simulink model "TST_EngPrt_PrtLimOvht"  (R2016b)
settings: Solver=FixedStepDiscrete  StartTime=0.0  StopTime=0.02  FixedStep=sampleTime  RelTol=1e-3
values from neighbouring files (symbols this model uses):
  testCase = 1    [initTST_EngPrt_PrtLimOvht_001.m]    (also in initTST_EngPrt_PrtLimOvht_002.m = 2; initTST_EngPrt_PrtLimOvht_003.m = 3; initTST_EngPrt_PrtLimOvht_004.m = 4; initTST_EngPrt_PrtLimOvht_005.m = 5)
libraries: simulink x21, UnitTest_Lib x10
(part 1 of 2)
settings Model: Creator=zhengjinyan  LastModifiedBy=zhengjinyan
settings DebuggingCC: SignalRangeChecking=error

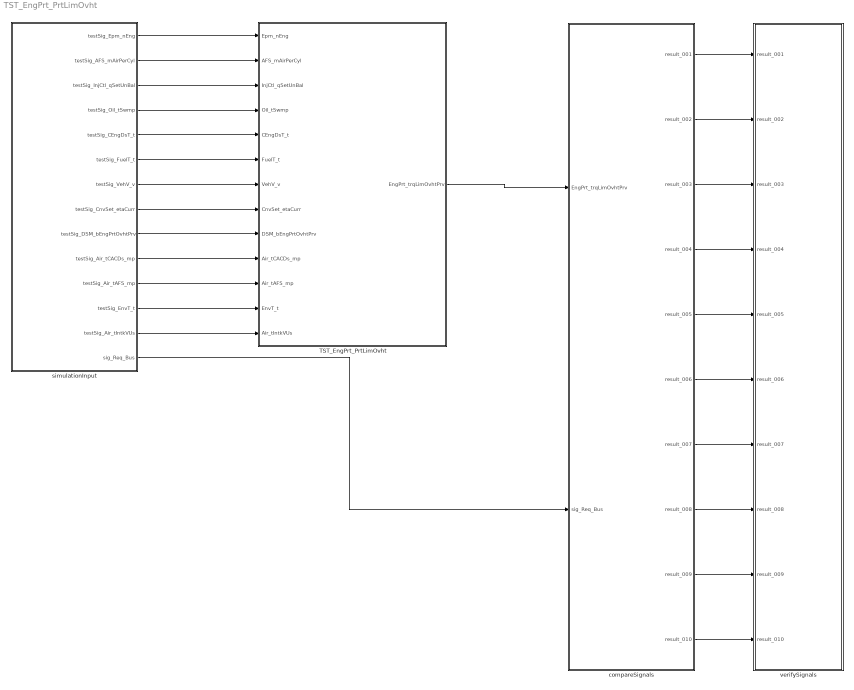
== system TST_EngPrt_PrtLimOvht ==
  TST_EngPrt_PrtLimOvht : Subsystem
  compareSignals : Subsystem
  simulationInput : Subsystem
  verifySignals : Subsystem
  wires:
  simulationInput/1(testSig_Epm_nEng) -> TST_EngPrt_PrtLimOvht/1(Epm_nEng)
  simulationInput/2(testSig_AFS_mAirPerCyl) -> TST_EngPrt_PrtLimOvht/2(AFS_mAirPerCyl)
  simulationInput/3(testSig_InjCtl_qSetUnBal) -> TST_EngPrt_PrtLimOvht/3(InjCtl_qSetUnBal)
  simulationInput/4(testSig_Oil_tSwmp) -> TST_EngPrt_PrtLimOvht/4(Oil_tSwmp)
  simulationInput/5(testSig_CEngDsT_t) -> TST_EngPrt_PrtLimOvht/5(CEngDsT_t)
  simulationInput/6(testSig_FuelT_t) -> TST_EngPrt_PrtLimOvht/6(FuelT_t)
  simulationInput/7(testSig_VehV_v) -> TST_EngPrt_PrtLimOvht/7(VehV_v)
  simulationInput/8(testSig_CnvSet_etaCurr) -> TST_EngPrt_PrtLimOvht/8(CnvSet_etaCurr)
  simulationInput/9(testSig_DSM_bEngPrtOvhtPrv) -> TST_EngPrt_PrtLimOvht/9(DSM_bEngPrtOvhtPrv)
  simulationInput/10(testSig_Air_tCACDs_mp) -> TST_EngPrt_PrtLimOvht/10(Air_tCACDs_mp)
  simulationInput/11(testSig_Air_tAFS_mp) -> TST_EngPrt_PrtLimOvht/11(Air_tAFS_mp)
  simulationInput/12(testSig_EnvT_t) -> TST_EngPrt_PrtLimOvht/12(EnvT_t)
  simulationInput/13(testSig_Air_tIntkVUs) -> TST_EngPrt_PrtLimOvht/13(Air_tIntkVUs)
  TST_EngPrt_PrtLimOvht/1(EngPrt_trqLimOvhtPrv) -> compareSignals/1(EngPrt_trqLimOvhtPrv)
  simulationInput/14(sig_Req_Bus) -> compareSignals/2(sig_Req_Bus)
  compareSignals/1(result_001) -> verifySignals/1(result_001)
  compareSignals/2(result_002) -> verifySignals/2(result_002)
  compareSignals/3(result_003) -> verifySignals/3(result_003)
  compareSignals/4(result_004) -> verifySignals/4(result_004)
  compareSignals/5(result_005) -> verifySignals/5(result_005)
  compareSignals/6(result_006) -> verifySignals/6(result_006)
  compareSignals/7(result_007) -> verifySignals/7(result_007)
  compareSignals/8(result_008) -> verifySignals/8(result_008)
  compareSignals/9(result_009) -> verifySignals/9(result_009)
  compareSignals/10(result_010) -> verifySignals/10(result_010)

== system TST_EngPrt_PrtLimOvht/TST_EngPrt_PrtLimOvht ==
  Epm_nEng : Inport
  AFS_mAirPerCyl : Inport  Port=2
  InjCtl_qSetUnBal : Inport  Port=3
  Oil_tSwmp : Inport  Port=4
  CEngDsT_t : Inport  Port=5
  FuelT_t : Inport  Port=6
  VehV_v : Inport  Port=7
  CnvSet_etaCurr : Inport  Port=8
  DSM_bEngPrtOvhtPrv : Inport  Port=9
  Air_tCACDs_mp : Inport  Port=10
  Air_tAFS_mp : Inport  Port=11
  EnvT_t : Inport  Port=12
  Air_tIntkVUs : Inport  Port=13
  EngPrt_PrtLimOvht : ModelReference  ModelNameDialog=EngPrt_PrtLimOvht  SimulationMode=Normal  ModelReferenceVersion=1.27  TriggerPortName=function  TriggerPortTriggerType=function-call  TriggerPortStatesWhenEnabling=held
  Function_Call : simulink/Ports & Subsystems/Function-Call Generator  sample_time=sampleTime  numberOfIterations=1
  EngPrt_trqLimOvhtPrv : Outport
  wires:
  Function_Call/1 -> EngPrt_PrtLimOvht/Trigger
  Epm_nEng/1 -> EngPrt_PrtLimOvht/1
  AFS_mAirPerCyl/1 -> EngPrt_PrtLimOvht/2
  InjCtl_qSetUnBal/1 -> EngPrt_PrtLimOvht/3
  Oil_tSwmp/1 -> EngPrt_PrtLimOvht/4
  CEngDsT_t/1 -> EngPrt_PrtLimOvht/5
  FuelT_t/1 -> EngPrt_PrtLimOvht/6
  VehV_v/1 -> EngPrt_PrtLimOvht/7
  CnvSet_etaCurr/1 -> EngPrt_PrtLimOvht/8
  DSM_bEngPrtOvhtPrv/1 -> EngPrt_PrtLimOvht/9
  Air_tCACDs_mp/1 -> EngPrt_PrtLimOvht/10
  Air_tAFS_mp/1 -> EngPrt_PrtLimOvht/11
  EnvT_t/1 -> EngPrt_PrtLimOvht/12
  Air_tIntkVUs/1 -> EngPrt_PrtLimOvht/13
  EngPrt_PrtLimOvht/1 -> EngPrt_trqLimOvhtPrv/1

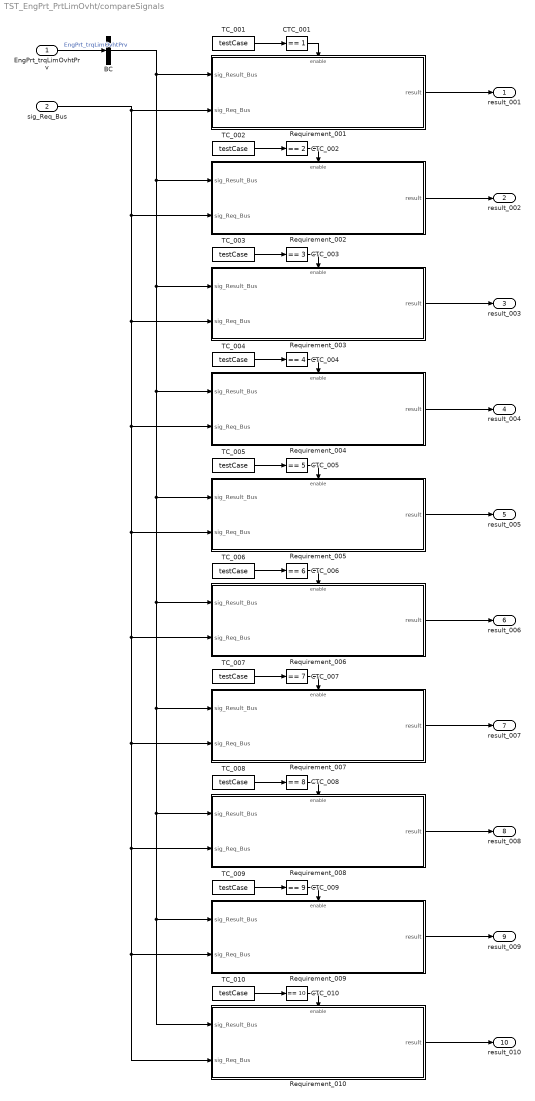
== system TST_EngPrt_PrtLimOvht/compareSignals ==
  EngPrt_trqLimOvhtPrv : Inport
  sig_Req_Bus : Inport  Port=2
  BC : BusCreator  Inputs=1
  CTC_001 : simulink/Logic and Bit Operations/Compare To Constant  relop===  const=1  OutDataTypeStr=boolean
  CTC_002 : simulink/Logic and Bit Operations/Compare To Constant  relop===  const=2  OutDataTypeStr=boolean
  CTC_003 : simulink/Logic and Bit Operations/Compare To Constant  relop===  const=3  OutDataTypeStr=boolean
  CTC_004 : simulink/Logic and Bit Operations/Compare To Constant  relop===  const=4  OutDataTypeStr=boolean
  CTC_005 : simulink/Logic and Bit Operations/Compare To Constant  relop===  const=5  OutDataTypeStr=boolean
  CTC_006 : simulink/Logic and Bit Operations/Compare To Constant  relop===  const=6  OutDataTypeStr=boolean
  CTC_007 : simulink/Logic and Bit Operations/Compare To Constant  relop===  const=7  OutDataTypeStr=boolean
  CTC_008 : simulink/Logic and Bit Operations/Compare To Constant  relop===  const=8  OutDataTypeStr=boolean
  CTC_009 : simulink/Logic and Bit Operations/Compare To Constant  relop===  const=9  OutDataTypeStr=boolean
  CTC_010 : simulink/Logic and Bit Operations/Compare To Constant  relop===  const=10  OutDataTypeStr=boolean
  Requirement_001 : Subsystem
  Requirement_002 : Subsystem
  Requirement_003 : Subsystem
  Requirement_004 : Subsystem
  Requirement_005 : Subsystem
  Requirement_006 : Subsystem
  Requirement_007 : Subsystem
  Requirement_008 : Subsystem
  Requirement_009 : Subsystem
  Requirement_010 : Subsystem
  TC_001 : Constant  Value=testCase
  TC_002 : Constant  Value=testCase
  TC_003 : Constant  Value=testCase
  TC_004 : Constant  Value=testCase
  TC_005 : Constant  Value=testCase
  TC_006 : Constant  Value=testCase
  TC_007 : Constant  Value=testCase
  TC_008 : Constant  Value=testCase
  TC_009 : Constant  Value=testCase
  TC_010 : Constant  Value=testCase
  result_001 : Outport
  result_002 : Outport  Port=2
  result_003 : Outport  Port=3
  result_004 : Outport  Port=4
  result_005 : Outport  Port=5
  result_006 : Outport  Port=6
  result_007 : Outport  Port=7
  result_008 : Outport  Port=8
  result_009 : Outport  Port=9
  result_010 : Outport  Port=10
  wires:
  EngPrt_trqLimOvhtPrv/1 -> BC/1  "EngPrt_trqLimOvhtPrv"
  TC_001/1 -> CTC_001/1
  CTC_001/1 -> Requirement_001/Enable
  sig_Req_Bus/1 -> Requirement_009/2(sig_Req_Bus), Requirement_010/2(sig_Req_Bus), Requirement_008/2(sig_Req_Bus), Requirement_007/2(sig_Req_Bus), Requirement_006/2(sig_Req_Bus), Requirement_005/2(sig_Req_Bus), Requirement_004/2(sig_Req_Bus), Requirement_003/2(sig_Req_Bus), Requirement_002/2(sig_Req_Bus), Requirement_001/2(sig_Req_Bus)
  BC/1 -> Requirement_009/1(sig_Result_Bus), Requirement_010/1(sig_Result_Bus), Requirement_008/1(sig_Result_Bus), Requirement_007/1(sig_Result_Bus), Requirement_006/1(sig_Result_Bus), Requirement_005/1(sig_Result_Bus), Requirement_004/1(sig_Result_Bus), Requirement_003/1(sig_Result_Bus), Requirement_002/1(sig_Result_Bus), Requirement_001/1(sig_Result_Bus)
  Requirement_001/1(result) -> result_001/1
  TC_002/1 -> CTC_002/1
  CTC_002/1 -> Requirement_002/Enable
  Requirement_002/1(result) -> result_002/1
  TC_003/1 -> CTC_003/1
  CTC_003/1 -> Requirement_003/Enable
  Requirement_003/1(result) -> result_003/1
  TC_004/1 -> CTC_004/1
  CTC_004/1 -> Requirement_004/Enable
  Requirement_004/1(result) -> result_004/1
  TC_005/1 -> CTC_005/1
  CTC_005/1 -> Requirement_005/Enable
  Requirement_005/1(result) -> result_005/1
  TC_006/1 -> CTC_006/1
  CTC_006/1 -> Requirement_006/Enable
  Requirement_006/1(result) -> result_006/1
  TC_007/1 -> CTC_007/1
  CTC_007/1 -> Requirement_007/Enable
  Requirement_007/1(result) -> result_007/1
  TC_008/1 -> CTC_008/1
  CTC_008/1 -> Requirement_008/Enable
  Requirement_008/1(result) -> result_008/1
  TC_009/1 -> CTC_009/1
  CTC_009/1 -> Requirement_009/Enable
  Requirement_009/1(result) -> result_009/1
  TC_010/1 -> CTC_010/1
  CTC_010/1 -> Requirement_010/Enable
  Requirement_010/1(result) -> result_010/1

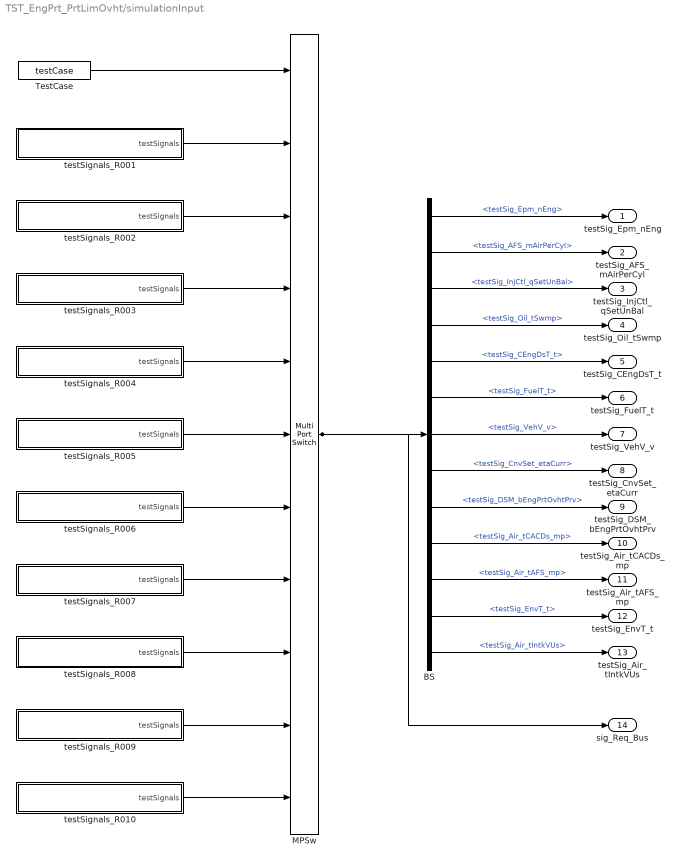
== system TST_EngPrt_PrtLimOvht/simulationInput ==
  BS : BusSelector  OutputSignals=testSig_Epm_nEng,testSig_AFS_mAirPerCyl,testSig_InjCtl_qSetUnBal,testSig_Oil_tSwmp,testSig_CEngDsT_t,testSig_FuelT_t,testSig_VehV_v,testSig_CnvSet_etaCurr,testSig_DSM_bEngPrtOvhtPrv,testSig_Air_tCACDs_mp,testSig_Air_tAFS_mp,testSig_EnvT_t,testSig_Air_tIntkVUs
  MPSw : MultiPortSwitch  Inputs=10  SaturateOnIntegerOverflow=on  InputSameDT=on
  TestCase : Constant  Value=testCase
  testSignals_R001 : Subsystem
  testSignals_R002 : Subsystem
  testSignals_R003 : Subsystem
  testSignals_R004 : Subsystem
  testSignals_R005 : Subsystem
  testSignals_R006 : Subsystem
  testSignals_R007 : Subsystem
  testSignals_R008 : Subsystem
  testSignals_R009 : Subsystem
  testSignals_R010 : Subsystem
  testSig_Epm_nEng : Outport
  testSig_AFS_mAirPerCyl : Outport  Port=2
  testSig_InjCtl_qSetUnBal : Outport  Port=3
  testSig_Oil_tSwmp : Outport  Port=4
  testSig_CEngDsT_t : Outport  Port=5
  testSig_FuelT_t : Outport  Port=6
  testSig_VehV_v : Outport  Port=7
  testSig_CnvSet_etaCurr : Outport  Port=8
  testSig_DSM_bEngPrtOvhtPrv : Outport  Port=9
  testSig_Air_tCACDs_mp : Outport  Port=10
  testSig_Air_tAFS_mp : Outport  Port=11
  testSig_EnvT_t : Outport  Port=12
  testSig_Air_tIntkVUs : Outport  Port=13
  sig_Req_Bus : Outport  Port=14
  wires:
  BS/1 -> testSig_Epm_nEng/1  "<testSig_Epm_nEng>"
  BS/2 -> testSig_AFS_mAirPerCyl/1  "<testSig_AFS_mAirPerCyl>"
  BS/3 -> testSig_InjCtl_qSetUnBal/1  "<testSig_InjCtl_qSetUnBal>"
  BS/4 -> testSig_Oil_tSwmp/1  "<testSig_Oil_tSwmp>"
  BS/5 -> testSig_CEngDsT_t/1  "<testSig_CEngDsT_t>"
  BS/6 -> testSig_FuelT_t/1  "<testSig_FuelT_t>"
  BS/7 -> testSig_VehV_v/1  "<testSig_VehV_v>"
  BS/8 -> testSig_CnvSet_etaCurr/1  "<testSig_CnvSet_etaCurr>"
  BS/9 -> testSig_DSM_bEngPrtOvhtPrv/1  "<testSig_DSM_bEngPrtOvhtPrv>"
  BS/10 -> testSig_Air_tCACDs_mp/1  "<testSig_Air_tCACDs_mp>"
  BS/11 -> testSig_Air_tAFS_mp/1  "<testSig_Air_tAFS_mp>"
  BS/12 -> testSig_EnvT_t/1  "<testSig_EnvT_t>"
  BS/13 -> testSig_Air_tIntkVUs/1  "<testSig_Air_tIntkVUs>"
  MPSw/1 -> BS/1, sig_Req_Bus/1
  TestCase/1 -> MPSw/1
  testSignals_R001/1(testSignals) -> MPSw/2
  testSignals_R002/1(testSignals) -> MPSw/3
  testSignals_R003/1(testSignals) -> MPSw/4
  testSignals_R004/1(testSignals) -> MPSw/5
  testSignals_R005/1(testSignals) -> MPSw/6
  testSignals_R006/1(testSignals) -> MPSw/7
  testSignals_R007/1(testSignals) -> MPSw/8
  testSignals_R008/1(testSignals) -> MPSw/9
  testSignals_R009/1(testSignals) -> MPSw/10
  testSignals_R010/1(testSignals) -> MPSw/11

== system TST_EngPrt_PrtLimOvht/verifySignals ==
  result_001 : Inport
  result_002 : Inport  Port=2
  result_003 : Inport  Port=3
  result_004 : Inport  Port=4
  result_005 : Inport  Port=5
  result_006 : Inport  Port=6
  result_007 : Inport  Port=7
  result_008 : Inport  Port=8
  result_009 : Inport  Port=9
  result_010 : Inport  Port=10
  Assertion_001 : Assertion  Enabled=off
  Assertion_002 : Assertion  Enabled=off
  Assertion_003 : Assertion  Enabled=off
  Assertion_004 : Assertion  Enabled=off
  Assertion_005 : Assertion  Enabled=off
  Assertion_006 : Assertion  Enabled=off
  Assertion_007 : Assertion  Enabled=off
  Assertion_008 : Assertion  Enabled=off
  Assertion_009 : Assertion  Enabled=off
  Assertion_010 : Assertion  Enabled=off
  wires:
  result_001/1 -> Assertion_001/1
  result_002/1 -> Assertion_002/1
  result_003/1 -> Assertion_003/1
  result_004/1 -> Assertion_004/1
  result_005/1 -> Assertion_005/1
  result_006/1 -> Assertion_006/1
  result_007/1 -> Assertion_007/1
  result_008/1 -> Assertion_008/1
  result_009/1 -> Assertion_009/1
  result_010/1 -> Assertion_010/1

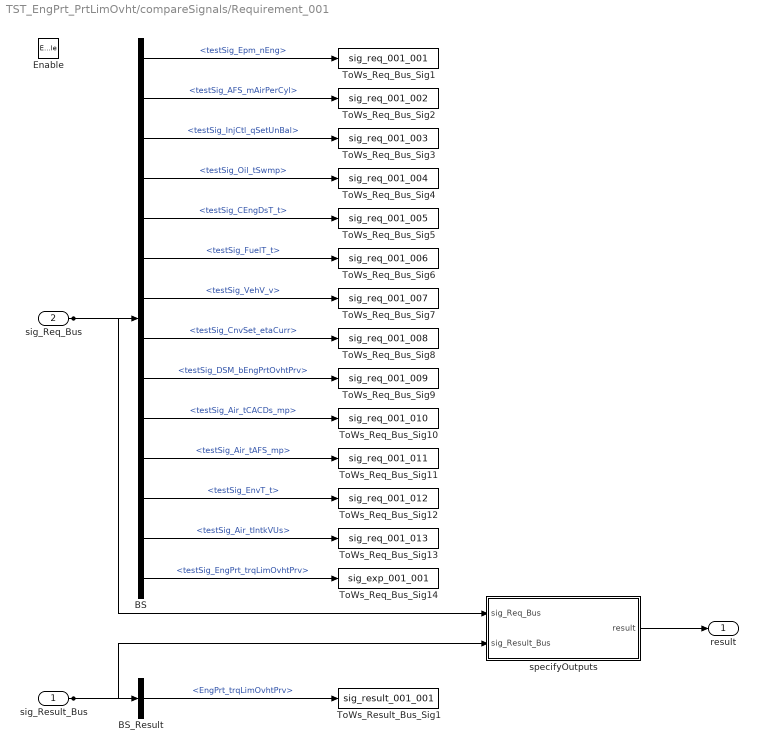
== system TST_EngPrt_PrtLimOvht/compareSignals/Requirement_001 ==
  sig_Result_Bus : Inport
  sig_Req_Bus : Inport  Port=2
  Enable : EnablePort
  BS : BusSelector  OutputSignals=testSig_Epm_nEng,testSig_AFS_mAirPerCyl,testSig_InjCtl_qSetUnBal,testSig_Oil_tSwmp,testSig_CEngDsT_t,testSig_FuelT_t,testSig_VehV_v,testSig_CnvSet_etaCurr,testSig_DSM_bEngPrtOvhtPrv,testSig_Air_tCACDs_mp,testSig_Air_tAFS_mp,testSig_EnvT_t,testSig_Air_tIntkVUs,testSig_EngPrt_trqLimOvhtPrv
  BS_Result : BusSelector  OutputSignals=EngPrt_trqLimOvhtPrv
  ToWs_Req_Bus_Sig1 : ToWorkspace  VariableName=sig_req_001_001  SaveFormat=Structure With Time
  ToWs_Req_Bus_Sig10 : ToWorkspace  VariableName=sig_req_001_010  SaveFormat=Structure With Time
  ToWs_Req_Bus_Sig11 : ToWorkspace  VariableName=sig_req_001_011  SaveFormat=Structure With Time
  ToWs_Req_Bus_Sig12 : ToWorkspace  VariableName=sig_req_001_012  SaveFormat=Structure With Time
  ToWs_Req_Bus_Sig13 : ToWorkspace  VariableName=sig_req_001_013  SaveFormat=Structure With Time
  ToWs_Req_Bus_Sig14 : ToWorkspace  VariableName=sig_exp_001_001  SaveFormat=Structure With Time
  ToWs_Req_Bus_Sig2 : ToWorkspace  VariableName=sig_req_001_002  SaveFormat=Structure With Time
  ToWs_Req_Bus_Sig3 : ToWorkspace  VariableName=sig_req_001_003  SaveFormat=Structure With Time
  ToWs_Req_Bus_Sig4 : ToWorkspace  VariableName=sig_req_001_004  SaveFormat=Structure With Time
  ToWs_Req_Bus_Sig5 : ToWorkspace  VariableName=sig_req_001_005  SaveFormat=Structure With Time
  ToWs_Req_Bus_Sig6 : ToWorkspace  VariableName=sig_req_001_006  SaveFormat=Structure With Time
  ToWs_Req_Bus_Sig7 : ToWorkspace  VariableName=sig_req_001_007  SaveFormat=Structure With Time
  ToWs_Req_Bus_Sig8 : ToWorkspace  VariableName=sig_req_001_008  SaveFormat=Structure With Time
  ToWs_Req_Bus_Sig9 : ToWorkspace  VariableName=sig_req_001_009  SaveFormat=Structure With Time
  ToWs_Result_Bus_Sig1 : ToWorkspace  VariableName=sig_result_001_001  SaveFormat=Structure With Time
  specifyOutputs : Subsystem
  result : Outport
  wires:
  sig_Req_Bus/1 -> BS/1, specifyOutputs/1(sig_Req_Bus)
  BS/1 -> ToWs_Req_Bus_Sig1/1  "<testSig_Epm_nEng>"
  BS/2 -> ToWs_Req_Bus_Sig2/1  "<testSig_AFS_mAirPerCyl>"
  BS/3 -> ToWs_Req_Bus_Sig3/1  "<testSig_InjCtl_qSetUnBal>"
  BS/4 -> ToWs_Req_Bus_Sig4/1  "<testSig_Oil_tSwmp>"
  BS/5 -> ToWs_Req_Bus_Sig5/1  "<testSig_CEngDsT_t>"
  BS/6 -> ToWs_Req_Bus_Sig6/1  "<testSig_FuelT_t>"
  BS/7 -> ToWs_Req_Bus_Sig7/1  "<testSig_VehV_v>"
  BS/8 -> ToWs_Req_Bus_Sig8/1  "<testSig_CnvSet_etaCurr>"
  BS/9 -> ToWs_Req_Bus_Sig9/1  "<testSig_DSM_bEngPrtOvhtPrv>"
  BS/10 -> ToWs_Req_Bus_Sig10/1  "<testSig_Air_tCACDs_mp>"
  BS/11 -> ToWs_Req_Bus_Sig11/1  "<testSig_Air_tAFS_mp>"
  BS/12 -> ToWs_Req_Bus_Sig12/1  "<testSig_EnvT_t>"
  BS/13 -> ToWs_Req_Bus_Sig13/1  "<testSig_Air_tIntkVUs>"
  BS/14 -> ToWs_Req_Bus_Sig14/1  "<testSig_EngPrt_trqLimOvhtPrv>"
  sig_Result_Bus/1 -> BS_Result/1, specifyOutputs/2(sig_Result_Bus)
  BS_Result/1 -> ToWs_Result_Bus_Sig1/1  "<EngPrt_trqLimOvhtPrv>"
  specifyOutputs/1(result) -> result/1

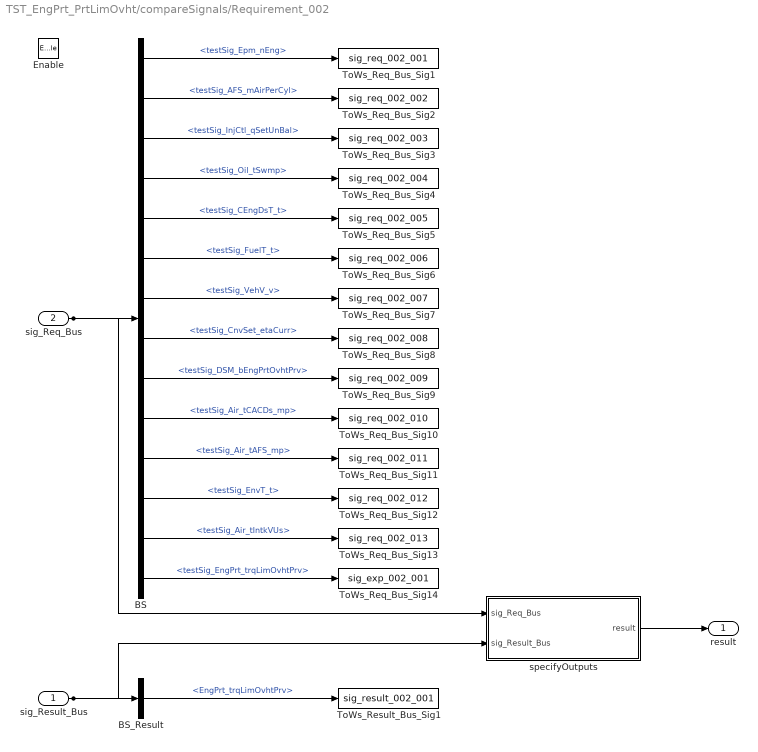
== system TST_EngPrt_PrtLimOvht/compareSignals/Requirement_002 ==
  sig_Result_Bus : Inport
  sig_Req_Bus : Inport  Port=2
  Enable : EnablePort
  BS : BusSelector  OutputSignals=testSig_Epm_nEng,testSig_AFS_mAirPerCyl,testSig_InjCtl_qSetUnBal,testSig_Oil_tSwmp,testSig_CEngDsT_t,testSig_FuelT_t,testSig_VehV_v,testSig_CnvSet_etaCurr,testSig_DSM_bEngPrtOvhtPrv,testSig_Air_tCACDs_mp,testSig_Air_tAFS_mp,testSig_EnvT_t,testSig_Air_tIntkVUs,testSig_EngPrt_trqLimOvhtPrv
  BS_Result : BusSelector  OutputSignals=EngPrt_trqLimOvhtPrv
  ToWs_Req_Bus_Sig1 : ToWorkspace  VariableName=sig_req_002_001  SaveFormat=Structure With Time
  ToWs_Req_Bus_Sig10 : ToWorkspace  VariableName=sig_req_002_010  SaveFormat=Structure With Time
  ToWs_Req_Bus_Sig11 : ToWorkspace  VariableName=sig_req_002_011  SaveFormat=Structure With Time
  ToWs_Req_Bus_Sig12 : ToWorkspace  VariableName=sig_req_002_012  SaveFormat=Structure With Time
  ToWs_Req_Bus_Sig13 : ToWorkspace  VariableName=sig_req_002_013  SaveFormat=Structure With Time
  ToWs_Req_Bus_Sig14 : ToWorkspace  VariableName=sig_exp_002_001  SaveFormat=Structure With Time
  ToWs_Req_Bus_Sig2 : ToWorkspace  VariableName=sig_req_002_002  SaveFormat=Structure With Time
  ToWs_Req_Bus_Sig3 : ToWorkspace  VariableName=sig_req_002_003  SaveFormat=Structure With Time
  ToWs_Req_Bus_Sig4 : ToWorkspace  VariableName=sig_req_002_004  SaveFormat=Structure With Time
  ToWs_Req_Bus_Sig5 : ToWorkspace  VariableName=sig_req_002_005  SaveFormat=Structure With Time
  ToWs_Req_Bus_Sig6 : ToWorkspace  VariableName=sig_req_002_006  SaveFormat=Structure With Time
  ToWs_Req_Bus_Sig7 : ToWorkspace  VariableName=sig_req_002_007  SaveFormat=Structure With Time
  ToWs_Req_Bus_Sig8 : ToWorkspace  VariableName=sig_req_002_008  SaveFormat=Structure With Time
  ToWs_Req_Bus_Sig9 : ToWorkspace  VariableName=sig_req_002_009  SaveFormat=Structure With Time
  ToWs_Result_Bus_Sig1 : ToWorkspace  VariableName=sig_result_002_001  SaveFormat=Structure With Time
  specifyOutputs : Subsystem
  result : Outport
  wires:
  sig_Req_Bus/1 -> BS/1, specifyOutputs/1(sig_Req_Bus)
  BS/1 -> ToWs_Req_Bus_Sig1/1  "<testSig_Epm_nEng>"
  BS/2 -> ToWs_Req_Bus_Sig2/1  "<testSig_AFS_mAirPerCyl>"
  BS/3 -> ToWs_Req_Bus_Sig3/1  "<testSig_InjCtl_qSetUnBal>"
  BS/4 -> ToWs_Req_Bus_Sig4/1  "<testSig_Oil_tSwmp>"
  BS/5 -> ToWs_Req_Bus_Sig5/1  "<testSig_CEngDsT_t>"
  BS/6 -> ToWs_Req_Bus_Sig6/1  "<testSig_FuelT_t>"
  BS/7 -> ToWs_Req_Bus_Sig7/1  "<testSig_VehV_v>"
  BS/8 -> ToWs_Req_Bus_Sig8/1  "<testSig_CnvSet_etaCurr>"
  BS/9 -> ToWs_Req_Bus_Sig9/1  "<testSig_DSM_bEngPrtOvhtPrv>"
  BS/10 -> ToWs_Req_Bus_Sig10/1  "<testSig_Air_tCACDs_mp>"
  BS/11 -> ToWs_Req_Bus_Sig11/1  "<testSig_Air_tAFS_mp>"
  BS/12 -> ToWs_Req_Bus_Sig12/1  "<testSig_EnvT_t>"
  BS/13 -> ToWs_Req_Bus_Sig13/1  "<testSig_Air_tIntkVUs>"
  BS/14 -> ToWs_Req_Bus_Sig14/1  "<testSig_EngPrt_trqLimOvhtPrv>"
  sig_Result_Bus/1 -> BS_Result/1, specifyOutputs/2(sig_Result_Bus)
  BS_Result/1 -> ToWs_Result_Bus_Sig1/1  "<EngPrt_trqLimOvhtPrv>"
  specifyOutputs/1(result) -> result/1

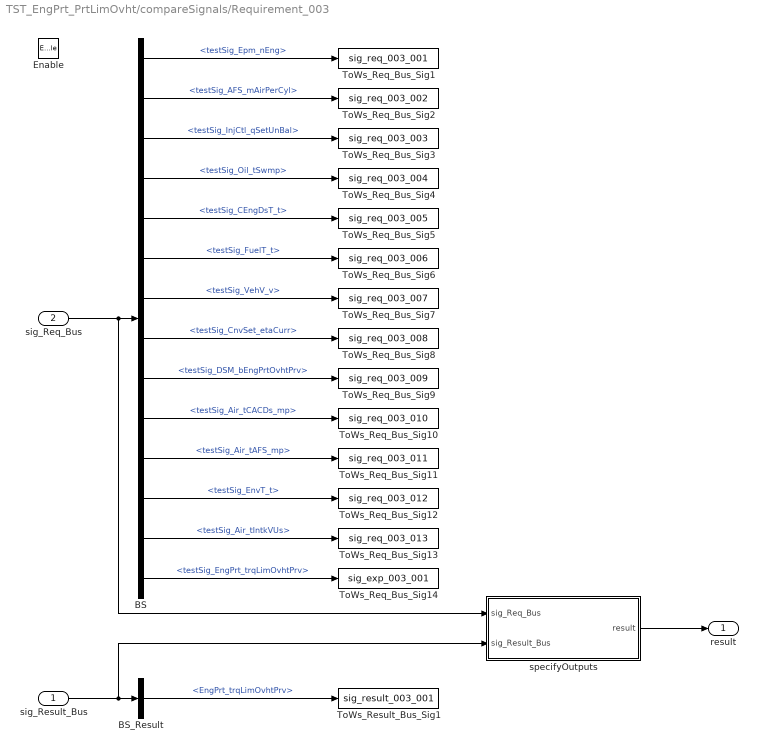
== system TST_EngPrt_PrtLimOvht/compareSignals/Requirement_003 ==
  sig_Result_Bus : Inport
  sig_Req_Bus : Inport  Port=2
  Enable : EnablePort
  BS : BusSelector  OutputSignals=testSig_Epm_nEng,testSig_AFS_mAirPerCyl,testSig_InjCtl_qSetUnBal,testSig_Oil_tSwmp,testSig_CEngDsT_t,testSig_FuelT_t,testSig_VehV_v,testSig_CnvSet_etaCurr,testSig_DSM_bEngPrtOvhtPrv,testSig_Air_tCACDs_mp,testSig_Air_tAFS_mp,testSig_EnvT_t,testSig_Air_tIntkVUs,testSig_EngPrt_trqLimOvhtPrv
  BS_Result : BusSelector  OutputSignals=EngPrt_trqLimOvhtPrv
  ToWs_Req_Bus_Sig1 : ToWorkspace  VariableName=sig_req_003_001  SaveFormat=Structure With Time
  ToWs_Req_Bus_Sig10 : ToWorkspace  VariableName=sig_req_003_010  SaveFormat=Structure With Time
  ToWs_Req_Bus_Sig11 : ToWorkspace  VariableName=sig_req_003_011  SaveFormat=Structure With Time
  ToWs_Req_Bus_Sig12 : ToWorkspace  VariableName=sig_req_003_012  SaveFormat=Structure With Time
  ToWs_Req_Bus_Sig13 : ToWorkspace  VariableName=sig_req_003_013  SaveFormat=Structure With Time
  ToWs_Req_Bus_Sig14 : ToWorkspace  VariableName=sig_exp_003_001  SaveFormat=Structure With Time
  ToWs_Req_Bus_Sig2 : ToWorkspace  VariableName=sig_req_003_002  SaveFormat=Structure With Time
  ToWs_Req_Bus_Sig3 : ToWorkspace  VariableName=sig_req_003_003  SaveFormat=Structure With Time
  ToWs_Req_Bus_Sig4 : ToWorkspace  VariableName=sig_req_003_004  SaveFormat=Structure With Time
  ToWs_Req_Bus_Sig5 : ToWorkspace  VariableName=sig_req_003_005  SaveFormat=Structure With Time
  ToWs_Req_Bus_Sig6 : ToWorkspace  VariableName=sig_req_003_006  SaveFormat=Structure With Time
  ToWs_Req_Bus_Sig7 : ToWorkspace  VariableName=sig_req_003_007  SaveFormat=Structure With Time
  ToWs_Req_Bus_Sig8 : ToWorkspace  VariableName=sig_req_003_008  SaveFormat=Structure With Time
  ToWs_Req_Bus_Sig9 : ToWorkspace  VariableName=sig_req_003_009  SaveFormat=Structure With Time
  ToWs_Result_Bus_Sig1 : ToWorkspace  VariableName=sig_result_003_001  SaveFormat=Structure With Time
  specifyOutputs : Subsystem
  result : Outport
  wires:
  sig_Req_Bus/1 -> BS/1, specifyOutputs/1(sig_Req_Bus)
  BS/1 -> ToWs_Req_Bus_Sig1/1  "<testSig_Epm_nEng>"
  BS/2 -> ToWs_Req_Bus_Sig2/1  "<testSig_AFS_mAirPerCyl>"
  BS/3 -> ToWs_Req_Bus_Sig3/1  "<testSig_InjCtl_qSetUnBal>"
  BS/4 -> ToWs_Req_Bus_Sig4/1  "<testSig_Oil_tSwmp>"
  BS/5 -> ToWs_Req_Bus_Sig5/1  "<testSig_CEngDsT_t>"
  BS/6 -> ToWs_Req_Bus_Sig6/1  "<testSig_FuelT_t>"
  BS/7 -> ToWs_Req_Bus_Sig7/1  "<testSig_VehV_v>"
  BS/8 -> ToWs_Req_Bus_Sig8/1  "<testSig_CnvSet_etaCurr>"
  BS/9 -> ToWs_Req_Bus_Sig9/1  "<testSig_DSM_bEngPrtOvhtPrv>"
  BS/10 -> ToWs_Req_Bus_Sig10/1  "<testSig_Air_tCACDs_mp>"
  BS/11 -> ToWs_Req_Bus_Sig11/1  "<testSig_Air_tAFS_mp>"
  BS/12 -> ToWs_Req_Bus_Sig12/1  "<testSig_EnvT_t>"
  BS/13 -> ToWs_Req_Bus_Sig13/1  "<testSig_Air_tIntkVUs>"
  BS/14 -> ToWs_Req_Bus_Sig14/1  "<testSig_EngPrt_trqLimOvhtPrv>"
  sig_Result_Bus/1 -> BS_Result/1, specifyOutputs/2(sig_Result_Bus)
  BS_Result/1 -> ToWs_Result_Bus_Sig1/1  "<EngPrt_trqLimOvhtPrv>"
  specifyOutputs/1(result) -> result/1

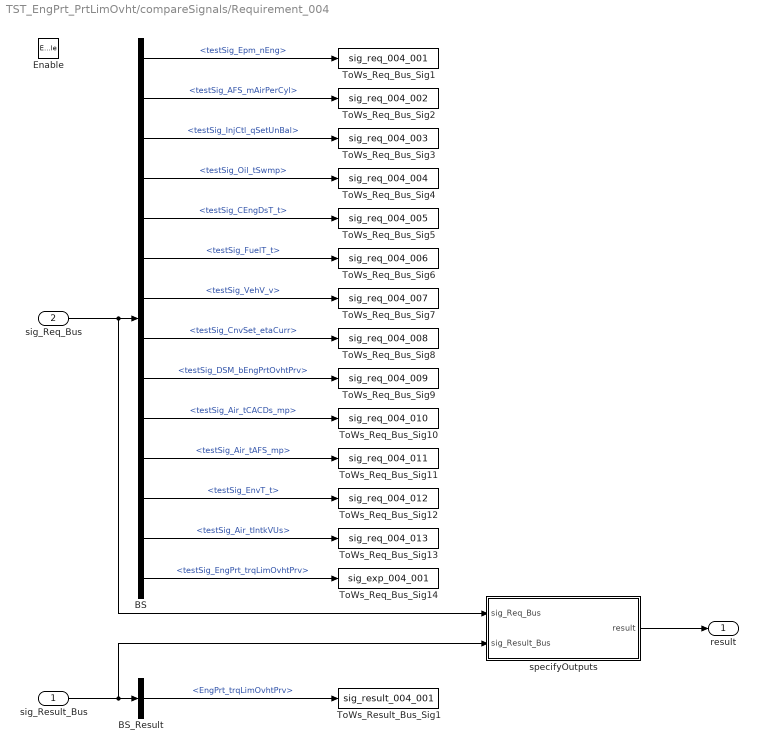
== system TST_EngPrt_PrtLimOvht/compareSignals/Requirement_004 ==
  sig_Result_Bus : Inport
  sig_Req_Bus : Inport  Port=2
  Enable : EnablePort
  BS : BusSelector  OutputSignals=testSig_Epm_nEng,testSig_AFS_mAirPerCyl,testSig_InjCtl_qSetUnBal,testSig_Oil_tSwmp,testSig_CEngDsT_t,testSig_FuelT_t,testSig_VehV_v,testSig_CnvSet_etaCurr,testSig_DSM_bEngPrtOvhtPrv,testSig_Air_tCACDs_mp,testSig_Air_tAFS_mp,testSig_EnvT_t,testSig_Air_tIntkVUs,testSig_EngPrt_trqLimOvhtPrv
  BS_Result : BusSelector  OutputSignals=EngPrt_trqLimOvhtPrv
  ToWs_Req_Bus_Sig1 : ToWorkspace  VariableName=sig_req_004_001  SaveFormat=Structure With Time
  ToWs_Req_Bus_Sig10 : ToWorkspace  VariableName=sig_req_004_010  SaveFormat=Structure With Time
  ToWs_Req_Bus_Sig11 : ToWorkspace  VariableName=sig_req_004_011  SaveFormat=Structure With Time
  ToWs_Req_Bus_Sig12 : ToWorkspace  VariableName=sig_req_004_012  SaveFormat=Structure With Time
  ToWs_Req_Bus_Sig13 : ToWorkspace  VariableName=sig_req_004_013  SaveFormat=Structure With Time
  ToWs_Req_Bus_Sig14 : ToWorkspace  VariableName=sig_exp_004_001  SaveFormat=Structure With Time
  ToWs_Req_Bus_Sig2 : ToWorkspace  VariableName=sig_req_004_002  SaveFormat=Structure With Time
  ToWs_Req_Bus_Sig3 : ToWorkspace  VariableName=sig_req_004_003  SaveFormat=Structure With Time
  ToWs_Req_Bus_Sig4 : ToWorkspace  VariableName=sig_req_004_004  SaveFormat=Structure With Time
  ToWs_Req_Bus_Sig5 : ToWorkspace  VariableName=sig_req_004_005  SaveFormat=Structure With Time
  ToWs_Req_Bus_Sig6 : ToWorkspace  VariableName=sig_req_004_006  SaveFormat=Structure With Time
  ToWs_Req_Bus_Sig7 : ToWorkspace  VariableName=sig_req_004_007  SaveFormat=Structure With Time
  ToWs_Req_Bus_Sig8 : ToWorkspace  VariableName=sig_req_004_008  SaveFormat=Structure With Time
  ToWs_Req_Bus_Sig9 : ToWorkspace  VariableName=sig_req_004_009  SaveFormat=Structure With Time
  ToWs_Result_Bus_Sig1 : ToWorkspace  VariableName=sig_result_004_001  SaveFormat=Structure With Time
  specifyOutputs : Subsystem
  result : Outport
  wires:
  sig_Req_Bus/1 -> BS/1, specifyOutputs/1(sig_Req_Bus)
  BS/1 -> ToWs_Req_Bus_Sig1/1  "<testSig_Epm_nEng>"
  BS/2 -> ToWs_Req_Bus_Sig2/1  "<testSig_AFS_mAirPerCyl>"
  BS/3 -> ToWs_Req_Bus_Sig3/1  "<testSig_InjCtl_qSetUnBal>"
  BS/4 -> ToWs_Req_Bus_Sig4/1  "<testSig_Oil_tSwmp>"
  BS/5 -> ToWs_Req_Bus_Sig5/1  "<testSig_CEngDsT_t>"
  BS/6 -> ToWs_Req_Bus_Sig6/1  "<testSig_FuelT_t>"
  BS/7 -> ToWs_Req_Bus_Sig7/1  "<testSig_VehV_v>"
  BS/8 -> ToWs_Req_Bus_Sig8/1  "<testSig_CnvSet_etaCurr>"
  BS/9 -> ToWs_Req_Bus_Sig9/1  "<testSig_DSM_bEngPrtOvhtPrv>"
  BS/10 -> ToWs_Req_Bus_Sig10/1  "<testSig_Air_tCACDs_mp>"
  BS/11 -> ToWs_Req_Bus_Sig11/1  "<testSig_Air_tAFS_mp>"
  BS/12 -> ToWs_Req_Bus_Sig12/1  "<testSig_EnvT_t>"
  BS/13 -> ToWs_Req_Bus_Sig13/1  "<testSig_Air_tIntkVUs>"
  BS/14 -> ToWs_Req_Bus_Sig14/1  "<testSig_EngPrt_trqLimOvhtPrv>"
  sig_Result_Bus/1 -> BS_Result/1, specifyOutputs/2(sig_Result_Bus)
  BS_Result/1 -> ToWs_Result_Bus_Sig1/1  "<EngPrt_trqLimOvhtPrv>"
  specifyOutputs/1(result) -> result/1

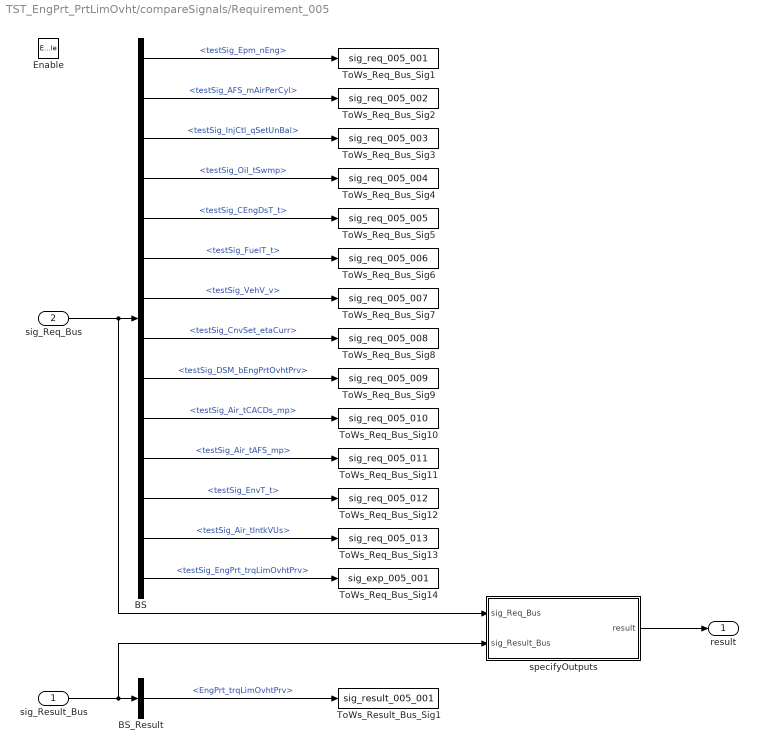
== system TST_EngPrt_PrtLimOvht/compareSignals/Requirement_005 ==
  sig_Result_Bus : Inport
  sig_Req_Bus : Inport  Port=2
  Enable : EnablePort
  BS : BusSelector  OutputSignals=testSig_Epm_nEng,testSig_AFS_mAirPerCyl,testSig_InjCtl_qSetUnBal,testSig_Oil_tSwmp,testSig_CEngDsT_t,testSig_FuelT_t,testSig_VehV_v,testSig_CnvSet_etaCurr,testSig_DSM_bEngPrtOvhtPrv,testSig_Air_tCACDs_mp,testSig_Air_tAFS_mp,testSig_EnvT_t,testSig_Air_tIntkVUs,testSig_EngPrt_trqLimOvhtPrv
  BS_Result : BusSelector  OutputSignals=EngPrt_trqLimOvhtPrv
  ToWs_Req_Bus_Sig1 : ToWorkspace  VariableName=sig_req_005_001  SaveFormat=Structure With Time
  ToWs_Req_Bus_Sig10 : ToWorkspace  VariableName=sig_req_005_010  SaveFormat=Structure With Time
  ToWs_Req_Bus_Sig11 : ToWorkspace  VariableName=sig_req_005_011  SaveFormat=Structure With Time
  ToWs_Req_Bus_Sig12 : ToWorkspace  VariableName=sig_req_005_012  SaveFormat=Structure With Time
  ToWs_Req_Bus_Sig13 : ToWorkspace  VariableName=sig_req_005_013  SaveFormat=Structure With Time
  ToWs_Req_Bus_Sig14 : ToWorkspace  VariableName=sig_exp_005_001  SaveFormat=Structure With Time
  ToWs_Req_Bus_Sig2 : ToWorkspace  VariableName=sig_req_005_002  SaveFormat=Structure With Time
  ToWs_Req_Bus_Sig3 : ToWorkspace  VariableName=sig_req_005_003  SaveFormat=Structure With Time
  ToWs_Req_Bus_Sig4 : ToWorkspace  VariableName=sig_req_005_004  SaveFormat=Structure With Time
  ToWs_Req_Bus_Sig5 : ToWorkspace  VariableName=sig_req_005_005  SaveFormat=Structure With Time
  ToWs_Req_Bus_Sig6 : ToWorkspace  VariableName=sig_req_005_006  SaveFormat=Structure With Time
  ToWs_Req_Bus_Sig7 : ToWorkspace  VariableName=sig_req_005_007  SaveFormat=Structure With Time
  ToWs_Req_Bus_Sig8 : ToWorkspace  VariableName=sig_req_005_008  SaveFormat=Structure With Time
  ToWs_Req_Bus_Sig9 : ToWorkspace  VariableName=sig_req_005_009  SaveFormat=Structure With Time
  ToWs_Result_Bus_Sig1 : ToWorkspace  VariableName=sig_result_005_001  SaveFormat=Structure With Time
  specifyOutputs : Subsystem
  result : Outport
  wires:
  sig_Req_Bus/1 -> BS/1, specifyOutputs/1(sig_Req_Bus)
  BS/1 -> ToWs_Req_Bus_Sig1/1  "<testSig_Epm_nEng>"
  BS/2 -> ToWs_Req_Bus_Sig2/1  "<testSig_AFS_mAirPerCyl>"
  BS/3 -> ToWs_Req_Bus_Sig3/1  "<testSig_InjCtl_qSetUnBal>"
  BS/4 -> ToWs_Req_Bus_Sig4/1  "<testSig_Oil_tSwmp>"
  BS/5 -> ToWs_Req_Bus_Sig5/1  "<testSig_CEngDsT_t>"
  BS/6 -> ToWs_Req_Bus_Sig6/1  "<testSig_FuelT_t>"
  BS/7 -> ToWs_Req_Bus_Sig7/1  "<testSig_VehV_v>"
  BS/8 -> ToWs_Req_Bus_Sig8/1  "<testSig_CnvSet_etaCurr>"
  BS/9 -> ToWs_Req_Bus_Sig9/1  "<testSig_DSM_bEngPrtOvhtPrv>"
  BS/10 -> ToWs_Req_Bus_Sig10/1  "<testSig_Air_tCACDs_mp>"
  BS/11 -> ToWs_Req_Bus_Sig11/1  "<testSig_Air_tAFS_mp>"
  BS/12 -> ToWs_Req_Bus_Sig12/1  "<testSig_EnvT_t>"
  BS/13 -> ToWs_Req_Bus_Sig13/1  "<testSig_Air_tIntkVUs>"
  BS/14 -> ToWs_Req_Bus_Sig14/1  "<testSig_EngPrt_trqLimOvhtPrv>"
  sig_Result_Bus/1 -> BS_Result/1, specifyOutputs/2(sig_Result_Bus)
  BS_Result/1 -> ToWs_Result_Bus_Sig1/1  "<EngPrt_trqLimOvhtPrv>"
  specifyOutputs/1(result) -> result/1

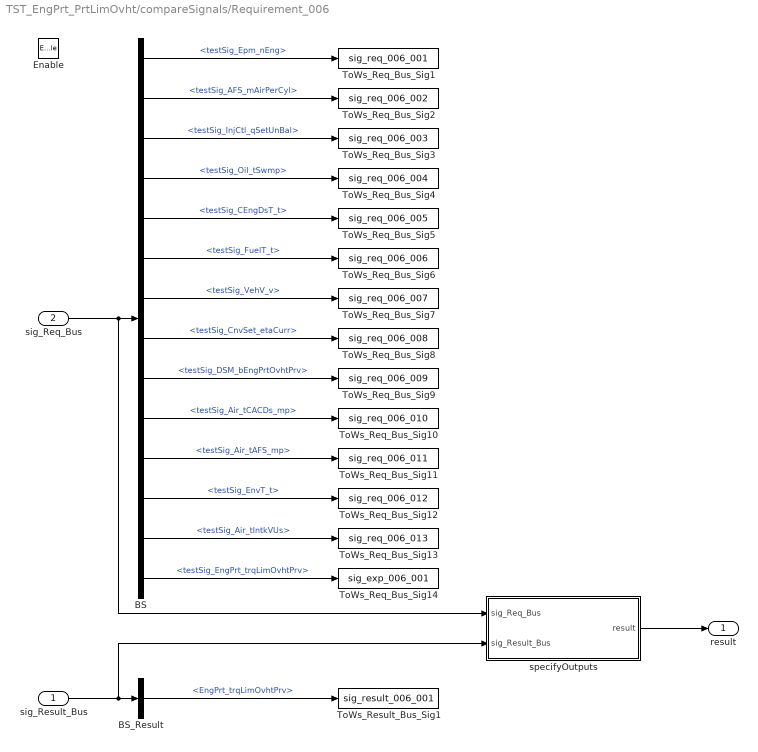
== system TST_EngPrt_PrtLimOvht/compareSignals/Requirement_006 ==
  sig_Result_Bus : Inport
  sig_Req_Bus : Inport  Port=2
  Enable : EnablePort
  BS : BusSelector  OutputSignals=testSig_Epm_nEng,testSig_AFS_mAirPerCyl,testSig_InjCtl_qSetUnBal,testSig_Oil_tSwmp,testSig_CEngDsT_t,testSig_FuelT_t,testSig_VehV_v,testSig_CnvSet_etaCurr,testSig_DSM_bEngPrtOvhtPrv,testSig_Air_tCACDs_mp,testSig_Air_tAFS_mp,testSig_EnvT_t,testSig_Air_tIntkVUs,testSig_EngPrt_trqLimOvhtPrv
  BS_Result : BusSelector  OutputSignals=EngPrt_trqLimOvhtPrv
  ToWs_Req_Bus_Sig1 : ToWorkspace  VariableName=sig_req_006_001  SaveFormat=Structure With Time
  ToWs_Req_Bus_Sig10 : ToWorkspace  VariableName=sig_req_006_010  SaveFormat=Structure With Time
  ToWs_Req_Bus_Sig11 : ToWorkspace  VariableName=sig_req_006_011  SaveFormat=Structure With Time
  ToWs_Req_Bus_Sig12 : ToWorkspace  VariableName=sig_req_006_012  SaveFormat=Structure With Time
  ToWs_Req_Bus_Sig13 : ToWorkspace  VariableName=sig_req_006_013  SaveFormat=Structure With Time
  ToWs_Req_Bus_Sig14 : ToWorkspace  VariableName=sig_exp_006_001  SaveFormat=Structure With Time
  ToWs_Req_Bus_Sig2 : ToWorkspace  VariableName=sig_req_006_002  SaveFormat=Structure With Time
  ToWs_Req_Bus_Sig3 : ToWorkspace  VariableName=sig_req_006_003  SaveFormat=Structure With Time
  ToWs_Req_Bus_Sig4 : ToWorkspace  VariableName=sig_req_006_004  SaveFormat=Structure With Time
  ToWs_Req_Bus_Sig5 : ToWorkspace  VariableName=sig_req_006_005  SaveFormat=Structure With Time
  ToWs_Req_Bus_Sig6 : ToWorkspace  VariableName=sig_req_006_006  SaveFormat=Structure With Time
  ToWs_Req_Bus_Sig7 : ToWorkspace  VariableName=sig_req_006_007  SaveFormat=Structure With Time
  ToWs_Req_Bus_Sig8 : ToWorkspace  VariableName=sig_req_006_008  SaveFormat=Structure With Time
  ToWs_Req_Bus_Sig9 : ToWorkspace  VariableName=sig_req_006_009  SaveFormat=Structure With Time
  ToWs_Result_Bus_Sig1 : ToWorkspace  VariableName=sig_result_006_001  SaveFormat=Structure With Time
  specifyOutputs : Subsystem
  result : Outport
  wires:
  sig_Req_Bus/1 -> BS/1, specifyOutputs/1(sig_Req_Bus)
  BS/1 -> ToWs_Req_Bus_Sig1/1  "<testSig_Epm_nEng>"
  BS/2 -> ToWs_Req_Bus_Sig2/1  "<testSig_AFS_mAirPerCyl>"
  BS/3 -> ToWs_Req_Bus_Sig3/1  "<testSig_InjCtl_qSetUnBal>"
  BS/4 -> ToWs_Req_Bus_Sig4/1  "<testSig_Oil_tSwmp>"
  BS/5 -> ToWs_Req_Bus_Sig5/1  "<testSig_CEngDsT_t>"
  BS/6 -> ToWs_Req_Bus_Sig6/1  "<testSig_FuelT_t>"
  BS/7 -> ToWs_Req_Bus_Sig7/1  "<testSig_VehV_v>"
  BS/8 -> ToWs_Req_Bus_Sig8/1  "<testSig_CnvSet_etaCurr>"
  BS/9 -> ToWs_Req_Bus_Sig9/1  "<testSig_DSM_bEngPrtOvhtPrv>"
  BS/10 -> ToWs_Req_Bus_Sig10/1  "<testSig_Air_tCACDs_mp>"
  BS/11 -> ToWs_Req_Bus_Sig11/1  "<testSig_Air_tAFS_mp>"
  BS/12 -> ToWs_Req_Bus_Sig12/1  "<testSig_EnvT_t>"
  BS/13 -> ToWs_Req_Bus_Sig13/1  "<testSig_Air_tIntkVUs>"
  BS/14 -> ToWs_Req_Bus_Sig14/1  "<testSig_EngPrt_trqLimOvhtPrv>"
  sig_Result_Bus/1 -> BS_Result/1, specifyOutputs/2(sig_Result_Bus)
  BS_Result/1 -> ToWs_Result_Bus_Sig1/1  "<EngPrt_trqLimOvhtPrv>"
  specifyOutputs/1(result) -> result/1

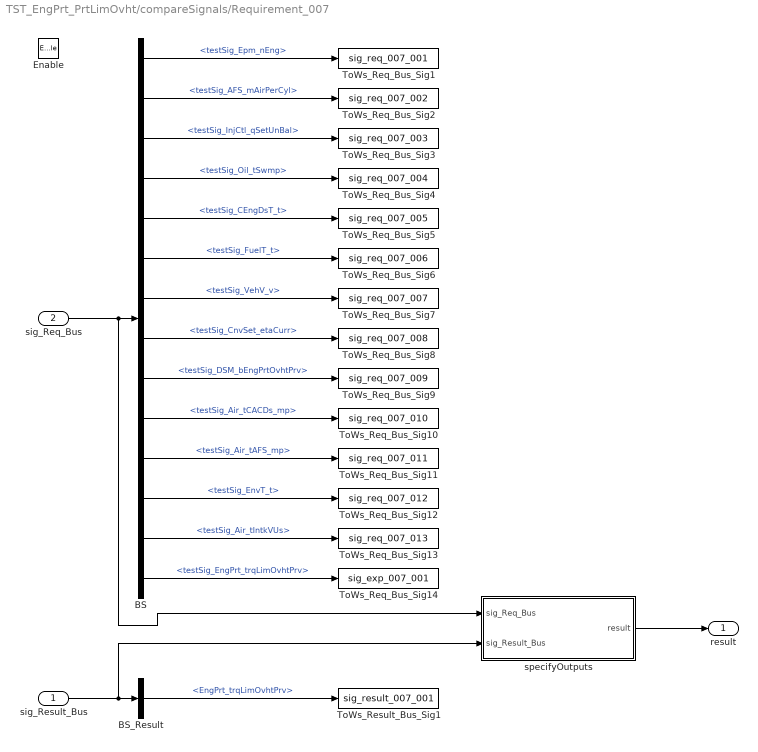
== system TST_EngPrt_PrtLimOvht/compareSignals/Requirement_007 ==
  sig_Result_Bus : Inport
  sig_Req_Bus : Inport  Port=2
  Enable : EnablePort
  BS : BusSelector  OutputSignals=testSig_Epm_nEng,testSig_AFS_mAirPerCyl,testSig_InjCtl_qSetUnBal,testSig_Oil_tSwmp,testSig_CEngDsT_t,testSig_FuelT_t,testSig_VehV_v,testSig_CnvSet_etaCurr,testSig_DSM_bEngPrtOvhtPrv,testSig_Air_tCACDs_mp,testSig_Air_tAFS_mp,testSig_EnvT_t,testSig_Air_tIntkVUs,testSig_EngPrt_trqLimOvhtPrv
  BS_Result : BusSelector  OutputSignals=EngPrt_trqLimOvhtPrv
  ToWs_Req_Bus_Sig1 : ToWorkspace  VariableName=sig_req_007_001  SaveFormat=Structure With Time
  ToWs_Req_Bus_Sig10 : ToWorkspace  VariableName=sig_req_007_010  SaveFormat=Structure With Time
  ToWs_Req_Bus_Sig11 : ToWorkspace  VariableName=sig_req_007_011  SaveFormat=Structure With Time
  ToWs_Req_Bus_Sig12 : ToWorkspace  VariableName=sig_req_007_012  SaveFormat=Structure With Time
  ToWs_Req_Bus_Sig13 : ToWorkspace  VariableName=sig_req_007_013  SaveFormat=Structure With Time
  ToWs_Req_Bus_Sig14 : ToWorkspace  VariableName=sig_exp_007_001  SaveFormat=Structure With Time
  ToWs_Req_Bus_Sig2 : ToWorkspace  VariableName=sig_req_007_002  SaveFormat=Structure With Time
  ToWs_Req_Bus_Sig3 : ToWorkspace  VariableName=sig_req_007_003  SaveFormat=Structure With Time
  ToWs_Req_Bus_Sig4 : ToWorkspace  VariableName=sig_req_007_004  SaveFormat=Structure With Time
  ToWs_Req_Bus_Sig5 : ToWorkspace  VariableName=sig_req_007_005  SaveFormat=Structure With Time
  ToWs_Req_Bus_Sig6 : ToWorkspace  VariableName=sig_req_007_006  SaveFormat=Structure With Time
  ToWs_Req_Bus_Sig7 : ToWorkspace  VariableName=sig_req_007_007  SaveFormat=Structure With Time
  ToWs_Req_Bus_Sig8 : ToWorkspace  VariableName=sig_req_007_008  SaveFormat=Structure With Time
  ToWs_Req_Bus_Sig9 : ToWorkspace  VariableName=sig_req_007_009  SaveFormat=Structure With Time
  ToWs_Result_Bus_Sig1 : ToWorkspace  VariableName=sig_result_007_001  SaveFormat=Structure With Time
  specifyOutputs : Subsystem
  result : Outport
  wires:
  sig_Req_Bus/1 -> BS/1, specifyOutputs/1(sig_Req_Bus)
  BS/1 -> ToWs_Req_Bus_Sig1/1  "<testSig_Epm_nEng>"
  BS/2 -> ToWs_Req_Bus_Sig2/1  "<testSig_AFS_mAirPerCyl>"
  BS/3 -> ToWs_Req_Bus_Sig3/1  "<testSig_InjCtl_qSetUnBal>"
  BS/4 -> ToWs_Req_Bus_Sig4/1  "<testSig_Oil_tSwmp>"
  BS/5 -> ToWs_Req_Bus_Sig5/1  "<testSig_CEngDsT_t>"
  BS/6 -> ToWs_Req_Bus_Sig6/1  "<testSig_FuelT_t>"
  BS/7 -> ToWs_Req_Bus_Sig7/1  "<testSig_VehV_v>"
  BS/8 -> ToWs_Req_Bus_Sig8/1  "<testSig_CnvSet_etaCurr>"
  BS/9 -> ToWs_Req_Bus_Sig9/1  "<testSig_DSM_bEngPrtOvhtPrv>"
  BS/10 -> ToWs_Req_Bus_Sig10/1  "<testSig_Air_tCACDs_mp>"
  BS/11 -> ToWs_Req_Bus_Sig11/1  "<testSig_Air_tAFS_mp>"
  BS/12 -> ToWs_Req_Bus_Sig12/1  "<testSig_EnvT_t>"
  BS/13 -> ToWs_Req_Bus_Sig13/1  "<testSig_Air_tIntkVUs>"
  BS/14 -> ToWs_Req_Bus_Sig14/1  "<testSig_EngPrt_trqLimOvhtPrv>"
  sig_Result_Bus/1 -> BS_Result/1, specifyOutputs/2(sig_Result_Bus)
  BS_Result/1 -> ToWs_Result_Bus_Sig1/1  "<EngPrt_trqLimOvhtPrv>"
  specifyOutputs/1(result) -> result/1

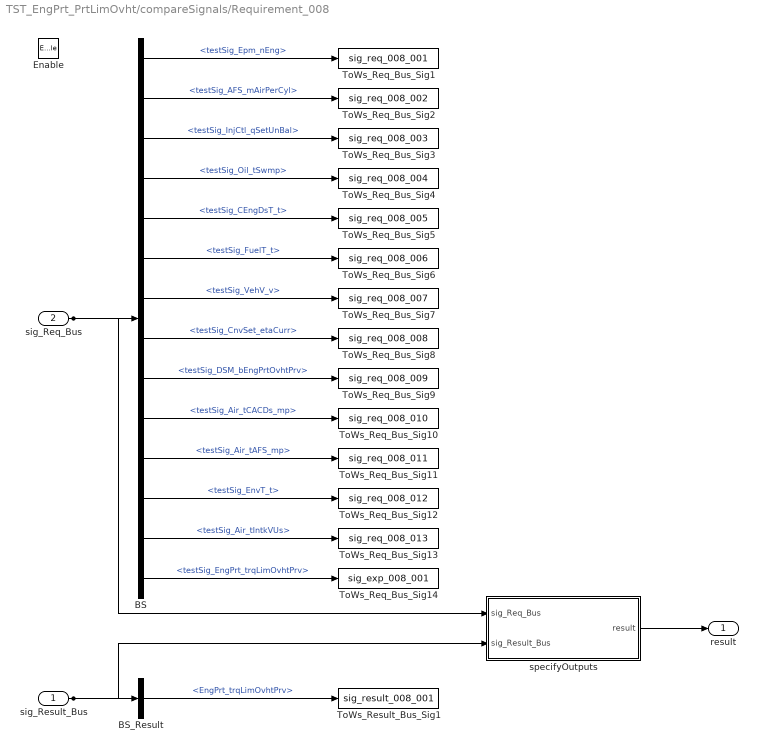
== system TST_EngPrt_PrtLimOvht/compareSignals/Requirement_008 ==
  sig_Result_Bus : Inport
  sig_Req_Bus : Inport  Port=2
  Enable : EnablePort
  BS : BusSelector  OutputSignals=testSig_Epm_nEng,testSig_AFS_mAirPerCyl,testSig_InjCtl_qSetUnBal,testSig_Oil_tSwmp,testSig_CEngDsT_t,testSig_FuelT_t,testSig_VehV_v,testSig_CnvSet_etaCurr,testSig_DSM_bEngPrtOvhtPrv,testSig_Air_tCACDs_mp,testSig_Air_tAFS_mp,testSig_EnvT_t,testSig_Air_tIntkVUs,testSig_EngPrt_trqLimOvhtPrv
  BS_Result : BusSelector  OutputSignals=EngPrt_trqLimOvhtPrv
  ToWs_Req_Bus_Sig1 : ToWorkspace  VariableName=sig_req_008_001  SaveFormat=Structure With Time
  ToWs_Req_Bus_Sig10 : ToWorkspace  VariableName=sig_req_008_010  SaveFormat=Structure With Time
  ToWs_Req_Bus_Sig11 : ToWorkspace  VariableName=sig_req_008_011  SaveFormat=Structure With Time
  ToWs_Req_Bus_Sig12 : ToWorkspace  VariableName=sig_req_008_012  SaveFormat=Structure With Time
  ToWs_Req_Bus_Sig13 : ToWorkspace  VariableName=sig_req_008_013  SaveFormat=Structure With Time
  ToWs_Req_Bus_Sig14 : ToWorkspace  VariableName=sig_exp_008_001  SaveFormat=Structure With Time
  ToWs_Req_Bus_Sig2 : ToWorkspace  VariableName=sig_req_008_002  SaveFormat=Structure With Time
  ToWs_Req_Bus_Sig3 : ToWorkspace  VariableName=sig_req_008_003  SaveFormat=Structure With Time
  ToWs_Req_Bus_Sig4 : ToWorkspace  VariableName=sig_req_008_004  SaveFormat=Structure With Time
  ToWs_Req_Bus_Sig5 : ToWorkspace  VariableName=sig_req_008_005  SaveFormat=Structure With Time
  ToWs_Req_Bus_Sig6 : ToWorkspace  VariableName=sig_req_008_006  SaveFormat=Structure With Time
  ToWs_Req_Bus_Sig7 : ToWorkspace  VariableName=sig_req_008_007  SaveFormat=Structure With Time
  ToWs_Req_Bus_Sig8 : ToWorkspace  VariableName=sig_req_008_008  SaveFormat=Structure With Time
  ToWs_Req_Bus_Sig9 : ToWorkspace  VariableName=sig_req_008_009  SaveFormat=Structure With Time
  ToWs_Result_Bus_Sig1 : ToWorkspace  VariableName=sig_result_008_001  SaveFormat=Structure With Time
  specifyOutputs : Subsystem
  result : Outport
  wires:
  sig_Req_Bus/1 -> BS/1, specifyOutputs/1(sig_Req_Bus)
  BS/1 -> ToWs_Req_Bus_Sig1/1  "<testSig_Epm_nEng>"
  BS/2 -> ToWs_Req_Bus_Sig2/1  "<testSig_AFS_mAirPerCyl>"
  BS/3 -> ToWs_Req_Bus_Sig3/1  "<testSig_InjCtl_qSetUnBal>"
  BS/4 -> ToWs_Req_Bus_Sig4/1  "<testSig_Oil_tSwmp>"
  BS/5 -> ToWs_Req_Bus_Sig5/1  "<testSig_CEngDsT_t>"
  BS/6 -> ToWs_Req_Bus_Sig6/1  "<testSig_FuelT_t>"
  BS/7 -> ToWs_Req_Bus_Sig7/1  "<testSig_VehV_v>"
  BS/8 -> ToWs_Req_Bus_Sig8/1  "<testSig_CnvSet_etaCurr>"
  BS/9 -> ToWs_Req_Bus_Sig9/1  "<testSig_DSM_bEngPrtOvhtPrv>"
  BS/10 -> ToWs_Req_Bus_Sig10/1  "<testSig_Air_tCACDs_mp>"
  BS/11 -> ToWs_Req_Bus_Sig11/1  "<testSig_Air_tAFS_mp>"
  BS/12 -> ToWs_Req_Bus_Sig12/1  "<testSig_EnvT_t>"
  BS/13 -> ToWs_Req_Bus_Sig13/1  "<testSig_Air_tIntkVUs>"
  BS/14 -> ToWs_Req_Bus_Sig14/1  "<testSig_EngPrt_trqLimOvhtPrv>"
  sig_Result_Bus/1 -> BS_Result/1, specifyOutputs/2(sig_Result_Bus)
  BS_Result/1 -> ToWs_Result_Bus_Sig1/1  "<EngPrt_trqLimOvhtPrv>"
  specifyOutputs/1(result) -> result/1

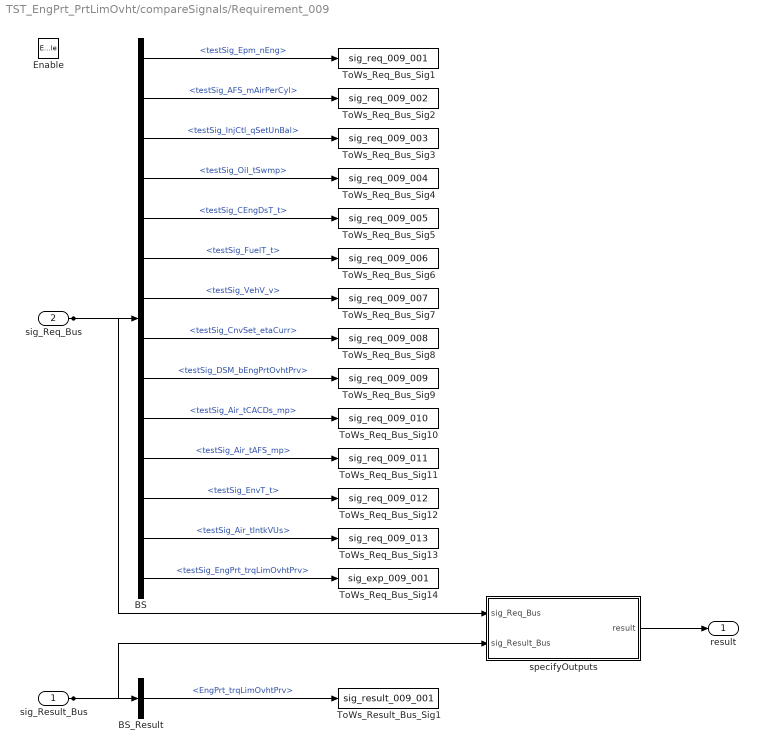
== system TST_EngPrt_PrtLimOvht/compareSignals/Requirement_009 ==
  sig_Result_Bus : Inport
  sig_Req_Bus : Inport  Port=2
  Enable : EnablePort
  BS : BusSelector  OutputSignals=testSig_Epm_nEng,testSig_AFS_mAirPerCyl,testSig_InjCtl_qSetUnBal,testSig_Oil_tSwmp,testSig_CEngDsT_t,testSig_FuelT_t,testSig_VehV_v,testSig_CnvSet_etaCurr,testSig_DSM_bEngPrtOvhtPrv,testSig_Air_tCACDs_mp,testSig_Air_tAFS_mp,testSig_EnvT_t,testSig_Air_tIntkVUs,testSig_EngPrt_trqLimOvhtPrv
  BS_Result : BusSelector  OutputSignals=EngPrt_trqLimOvhtPrv
  ToWs_Req_Bus_Sig1 : ToWorkspace  VariableName=sig_req_009_001  SaveFormat=Structure With Time
  ToWs_Req_Bus_Sig10 : ToWorkspace  VariableName=sig_req_009_010  SaveFormat=Structure With Time
  ToWs_Req_Bus_Sig11 : ToWorkspace  VariableName=sig_req_009_011  SaveFormat=Structure With Time
  ToWs_Req_Bus_Sig12 : ToWorkspace  VariableName=sig_req_009_012  SaveFormat=Structure With Time
  ToWs_Req_Bus_Sig13 : ToWorkspace  VariableName=sig_req_009_013  SaveFormat=Structure With Time
  ToWs_Req_Bus_Sig14 : ToWorkspace  VariableName=sig_exp_009_001  SaveFormat=Structure With Time
  ToWs_Req_Bus_Sig2 : ToWorkspace  VariableName=sig_req_009_002  SaveFormat=Structure With Time
  ToWs_Req_Bus_Sig3 : ToWorkspace  VariableName=sig_req_009_003  SaveFormat=Structure With Time
  ToWs_Req_Bus_Sig4 : ToWorkspace  VariableName=sig_req_009_004  SaveFormat=Structure With Time
  ToWs_Req_Bus_Sig5 : ToWorkspace  VariableName=sig_req_009_005  SaveFormat=Structure With Time
  ToWs_Req_Bus_Sig6 : ToWorkspace  VariableName=sig_req_009_006  SaveFormat=Structure With Time
  ToWs_Req_Bus_Sig7 : ToWorkspace  VariableName=sig_req_009_007  SaveFormat=Structure With Time
  ToWs_Req_Bus_Sig8 : ToWorkspace  VariableName=sig_req_009_008  SaveFormat=Structure With Time
  ToWs_Req_Bus_Sig9 : ToWorkspace  VariableName=sig_req_009_009  SaveFormat=Structure With Time
  ToWs_Result_Bus_Sig1 : ToWorkspace  VariableName=sig_result_009_001  SaveFormat=Structure With Time
  specifyOutputs : Subsystem
  result : Outport
  wires:
  sig_Req_Bus/1 -> BS/1, specifyOutputs/1(sig_Req_Bus)
  BS/1 -> ToWs_Req_Bus_Sig1/1  "<testSig_Epm_nEng>"
  BS/2 -> ToWs_Req_Bus_Sig2/1  "<testSig_AFS_mAirPerCyl>"
  BS/3 -> ToWs_Req_Bus_Sig3/1  "<testSig_InjCtl_qSetUnBal>"
  BS/4 -> ToWs_Req_Bus_Sig4/1  "<testSig_Oil_tSwmp>"
  BS/5 -> ToWs_Req_Bus_Sig5/1  "<testSig_CEngDsT_t>"
  BS/6 -> ToWs_Req_Bus_Sig6/1  "<testSig_FuelT_t>"
  BS/7 -> ToWs_Req_Bus_Sig7/1  "<testSig_VehV_v>"
  BS/8 -> ToWs_Req_Bus_Sig8/1  "<testSig_CnvSet_etaCurr>"
  BS/9 -> ToWs_Req_Bus_Sig9/1  "<testSig_DSM_bEngPrtOvhtPrv>"
  BS/10 -> ToWs_Req_Bus_Sig10/1  "<testSig_Air_tCACDs_mp>"
  BS/11 -> ToWs_Req_Bus_Sig11/1  "<testSig_Air_tAFS_mp>"
  BS/12 -> ToWs_Req_Bus_Sig12/1  "<testSig_EnvT_t>"
  BS/13 -> ToWs_Req_Bus_Sig13/1  "<testSig_Air_tIntkVUs>"
  BS/14 -> ToWs_Req_Bus_Sig14/1  "<testSig_EngPrt_trqLimOvhtPrv>"
  sig_Result_Bus/1 -> BS_Result/1, specifyOutputs/2(sig_Result_Bus)
  BS_Result/1 -> ToWs_Result_Bus_Sig1/1  "<EngPrt_trqLimOvhtPrv>"
  specifyOutputs/1(result) -> result/1

== system TST_EngPrt_PrtLimOvht/compareSignals/Requirement_010 ==
  sig_Result_Bus : Inport
  sig_Req_Bus : Inport  Port=2
  Enable : EnablePort
  BS : BusSelector  OutputSignals=testSig_Epm_nEng,testSig_AFS_mAirPerCyl,testSig_InjCtl_qSetUnBal,testSig_Oil_tSwmp,testSig_CEngDsT_t,testSig_FuelT_t,testSig_VehV_v,testSig_CnvSet_etaCurr,testSig_DSM_bEngPrtOvhtPrv,testSig_Air_tCACDs_mp,testSig_Air_tAFS_mp,testSig_EnvT_t,testSig_Air_tIntkVUs,testSig_EngPrt_trqLimOvhtPrv
  BS_Result : BusSelector  OutputSignals=EngPrt_trqLimOvhtPrv
  ToWs_Req_Bus_Sig1 : ToWorkspace  VariableName=sig_req_010_001  SaveFormat=Structure With Time
  ToWs_Req_Bus_Sig10 : ToWorkspace  VariableName=sig_req_010_010  SaveFormat=Structure With Time
  ToWs_Req_Bus_Sig11 : ToWorkspace  VariableName=sig_req_010_011  SaveFormat=Structure With Time
  ToWs_Req_Bus_Sig12 : ToWorkspace  VariableName=sig_req_010_012  SaveFormat=Structure With Time
  ToWs_Req_Bus_Sig13 : ToWorkspace  VariableName=sig_req_010_013  SaveFormat=Structure With Time
  ToWs_Req_Bus_Sig14 : ToWorkspace  VariableName=sig_exp_010_001  SaveFormat=Structure With Time
  ToWs_Req_Bus_Sig2 : ToWorkspace  VariableName=sig_req_010_002  SaveFormat=Structure With Time
  ToWs_Req_Bus_Sig3 : ToWorkspace  VariableName=sig_req_010_003  SaveFormat=Structure With Time
  ToWs_Req_Bus_Sig4 : ToWorkspace  VariableName=sig_req_010_004  SaveFormat=Structure With Time
  ToWs_Req_Bus_Sig5 : ToWorkspace  VariableName=sig_req_010_005  SaveFormat=Structure With Time
  ToWs_Req_Bus_Sig6 : ToWorkspace  VariableName=sig_req_010_006  SaveFormat=Structure With Time
  ToWs_Req_Bus_Sig7 : ToWorkspace  VariableName=sig_req_010_007  SaveFormat=Structure With Time
  ToWs_Req_Bus_Sig8 : ToWorkspace  VariableName=sig_req_010_008  SaveFormat=Structure With Time
  ToWs_Req_Bus_Sig9 : ToWorkspace  VariableName=sig_req_010_009  SaveFormat=Structure With Time
  ToWs_Result_Bus_Sig1 : ToWorkspace  VariableName=sig_result_010_001  SaveFormat=Structure With Time
  specifyOutputs : Subsystem
  result : Outport
  wires:
  sig_Req_Bus/1 -> BS/1, specifyOutputs/1(sig_Req_Bus)
  BS/1 -> ToWs_Req_Bus_Sig1/1  "<testSig_Epm_nEng>"
  BS/2 -> ToWs_Req_Bus_Sig2/1  "<testSig_AFS_mAirPerCyl>"
  BS/3 -> ToWs_Req_Bus_Sig3/1  "<testSig_InjCtl_qSetUnBal>"
  BS/4 -> ToWs_Req_Bus_Sig4/1  "<testSig_Oil_tSwmp>"
  BS/5 -> ToWs_Req_Bus_Sig5/1  "<testSig_CEngDsT_t>"
  BS/6 -> ToWs_Req_Bus_Sig6/1  "<testSig_FuelT_t>"
  BS/7 -> ToWs_Req_Bus_Sig7/1  "<testSig_VehV_v>"
  BS/8 -> ToWs_Req_Bus_Sig8/1  "<testSig_CnvSet_etaCurr>"
  BS/9 -> ToWs_Req_Bus_Sig9/1  "<testSig_DSM_bEngPrtOvhtPrv>"
  BS/10 -> ToWs_Req_Bus_Sig10/1  "<testSig_Air_tCACDs_mp>"
  BS/11 -> ToWs_Req_Bus_Sig11/1  "<testSig_Air_tAFS_mp>"
  BS/12 -> ToWs_Req_Bus_Sig12/1  "<testSig_EnvT_t>"
  BS/13 -> ToWs_Req_Bus_Sig13/1  "<testSig_Air_tIntkVUs>"
  BS/14 -> ToWs_Req_Bus_Sig14/1  "<testSig_EngPrt_trqLimOvhtPrv>"
  sig_Result_Bus/1 -> BS_Result/1, specifyOutputs/2(sig_Result_Bus)
  BS_Result/1 -> ToWs_Result_Bus_Sig1/1  "<EngPrt_trqLimOvhtPrv>"
  specifyOutputs/1(result) -> result/1

== system TST_EngPrt_PrtLimOvht/simulationInput/testSignals_R001 ==
  BC : BusCreator  Inputs=14
  spec_AFS_mAirPerCyl : FromWorkspace  VariableName=testSig_AFS_mAirPerCyl  Interpolate=off  OutputAfterFinalValue=Holding final value
  spec_Air_tAFS_mp : FromWorkspace  VariableName=testSig_Air_tAFS_mp  Interpolate=off  OutputAfterFinalValue=Holding final value
  spec_Air_tCACDs_mp : FromWorkspace  VariableName=testSig_Air_tCACDs_mp  Interpolate=off  OutputAfterFinalValue=Holding final value
  spec_Air_tIntkVUs : FromWorkspace  VariableName=testSig_Air_tIntkVUs  Interpolate=off  OutputAfterFinalValue=Holding final value
  spec_CEngDsT_t : FromWorkspace  VariableName=testSig_CEngDsT_t  Interpolate=off  OutputAfterFinalValue=Holding final value
  spec_CnvSet_etaCurr : FromWorkspace  VariableName=testSig_CnvSet_etaCurr  Interpolate=off  OutputAfterFinalValue=Holding final value
  spec_DSM_bEngPrtOvhtPrv : FromWorkspace  VariableName=testSig_DSM_bEngPrtOvhtPrv  Interpolate=off  OutputAfterFinalValue=Holding final value
  spec_EngPrt_trqLimOvhtPrv : FromWorkspace  VariableName=testSig_EngPrt_trqLimOvhtPrv  Interpolate=off  OutputAfterFinalValue=Holding final value
  spec_EnvT_t : FromWorkspace  VariableName=testSig_EnvT_t  Interpolate=off  OutputAfterFinalValue=Holding final value
  spec_Epm_nEng : FromWorkspace  VariableName=testSig_Epm_nEng  Interpolate=off  OutputAfterFinalValue=Holding final value
  spec_FuelT_t : FromWorkspace  VariableName=testSig_FuelT_t  Interpolate=off  OutputAfterFinalValue=Holding final value
  spec_InjCtl_qSetUnBal : FromWorkspace  VariableName=testSig_InjCtl_qSetUnBal  Interpolate=off  OutputAfterFinalValue=Holding final value
  spec_Oil_tSwmp : FromWorkspace  VariableName=testSig_Oil_tSwmp  Interpolate=off  OutputAfterFinalValue=Holding final value
  spec_VehV_v : FromWorkspace  VariableName=testSig_VehV_v  Interpolate=off  OutputAfterFinalValue=Holding final value
  testSignals : Outport
  wires:
  BC/1 -> testSignals/1
  spec_Epm_nEng/1 -> BC/1  "testSig_Epm_nEng"
  spec_AFS_mAirPerCyl/1 -> BC/2  "testSig_AFS_mAirPerCyl"
  spec_InjCtl_qSetUnBal/1 -> BC/3  "testSig_InjCtl_qSetUnBal"
  spec_Oil_tSwmp/1 -> BC/4  "testSig_Oil_tSwmp"
  spec_CEngDsT_t/1 -> BC/5  "testSig_CEngDsT_t"
  spec_FuelT_t/1 -> BC/6  "testSig_FuelT_t"
  spec_VehV_v/1 -> BC/7  "testSig_VehV_v"
  spec_CnvSet_etaCurr/1 -> BC/8  "testSig_CnvSet_etaCurr"
  spec_DSM_bEngPrtOvhtPrv/1 -> BC/9  "testSig_DSM_bEngPrtOvhtPrv"
  spec_Air_tCACDs_mp/1 -> BC/10  "testSig_Air_tCACDs_mp"
  spec_Air_tAFS_mp/1 -> BC/11  "testSig_Air_tAFS_mp"
  spec_EnvT_t/1 -> BC/12  "testSig_EnvT_t"
  spec_Air_tIntkVUs/1 -> BC/13  "testSig_Air_tIntkVUs"
  spec_EngPrt_trqLimOvhtPrv/1 -> BC/14  "testSig_EngPrt_trqLimOvhtPrv"

== system TST_EngPrt_PrtLimOvht/simulationInput/testSignals_R002 ==
  BC : BusCreator  Inputs=14
  spec_AFS_mAirPerCyl : FromWorkspace  VariableName=testSig_AFS_mAirPerCyl  Interpolate=off  OutputAfterFinalValue=Holding final value
  spec_Air_tAFS_mp : FromWorkspace  VariableName=testSig_Air_tAFS_mp  Interpolate=off  OutputAfterFinalValue=Holding final value
  spec_Air_tCACDs_mp : FromWorkspace  VariableName=testSig_Air_tCACDs_mp  Interpolate=off  OutputAfterFinalValue=Holding final value
  spec_Air_tIntkVUs : FromWorkspace  VariableName=testSig_Air_tIntkVUs  Interpolate=off  OutputAfterFinalValue=Holding final value
  spec_CEngDsT_t : FromWorkspace  VariableName=testSig_CEngDsT_t  Interpolate=off  OutputAfterFinalValue=Holding final value
  spec_CnvSet_etaCurr : FromWorkspace  VariableName=testSig_CnvSet_etaCurr  Interpolate=off  OutputAfterFinalValue=Holding final value
  spec_DSM_bEngPrtOvhtPrv : FromWorkspace  VariableName=testSig_DSM_bEngPrtOvhtPrv  Interpolate=off  OutputAfterFinalValue=Holding final value
  spec_EngPrt_trqLimOvhtPrv : FromWorkspace  VariableName=testSig_EngPrt_trqLimOvhtPrv  Interpolate=off  OutputAfterFinalValue=Holding final value
  spec_EnvT_t : FromWorkspace  VariableName=testSig_EnvT_t  Interpolate=off  OutputAfterFinalValue=Holding final value
  spec_Epm_nEng : FromWorkspace  VariableName=testSig_Epm_nEng  Interpolate=off  OutputAfterFinalValue=Holding final value
  spec_FuelT_t : FromWorkspace  VariableName=testSig_FuelT_t  Interpolate=off  OutputAfterFinalValue=Holding final value
  spec_InjCtl_qSetUnBal : FromWorkspace  VariableName=testSig_InjCtl_qSetUnBal  Interpolate=off  OutputAfterFinalValue=Holding final value
  spec_Oil_tSwmp : FromWorkspace  VariableName=testSig_Oil_tSwmp  Interpolate=off  OutputAfterFinalValue=Holding final value
  spec_VehV_v : FromWorkspace  VariableName=testSig_VehV_v  Interpolate=off  OutputAfterFinalValue=Holding final value
  testSignals : Outport
  wires:
  BC/1 -> testSignals/1
  spec_Epm_nEng/1 -> BC/1  "testSig_Epm_nEng"
  spec_AFS_mAirPerCyl/1 -> BC/2  "testSig_AFS_mAirPerCyl"
  spec_InjCtl_qSetUnBal/1 -> BC/3  "testSig_InjCtl_qSetUnBal"
  spec_Oil_tSwmp/1 -> BC/4  "testSig_Oil_tSwmp"
  spec_CEngDsT_t/1 -> BC/5  "testSig_CEngDsT_t"
  spec_FuelT_t/1 -> BC/6  "testSig_FuelT_t"
  spec_VehV_v/1 -> BC/7  "testSig_VehV_v"
  spec_CnvSet_etaCurr/1 -> BC/8  "testSig_CnvSet_etaCurr"
  spec_DSM_bEngPrtOvhtPrv/1 -> BC/9  "testSig_DSM_bEngPrtOvhtPrv"
  spec_Air_tCACDs_mp/1 -> BC/10  "testSig_Air_tCACDs_mp"
  spec_Air_tAFS_mp/1 -> BC/11  "testSig_Air_tAFS_mp"
  spec_EnvT_t/1 -> BC/12  "testSig_EnvT_t"
  spec_Air_tIntkVUs/1 -> BC/13  "testSig_Air_tIntkVUs"
  spec_EngPrt_trqLimOvhtPrv/1 -> BC/14  "testSig_EngPrt_trqLimOvhtPrv"
